simulink model "BbIb_parameter_estimation"  (R2022b)
settings: Solver=VariableStepAuto  StartTime=0.0  StopTime=25  MaxStep=0.005  RelTol=1e-3
values from neighbouring files (symbols this model uses):
  Bb = 0.00132333752617    [BbNew.mat]    (also in BbStiction.mat = 0.000317013532792; parameters.m = 0.000992; parametersDeadZone.m = 0.0001)
  Ib = 0.000954747737791    [IbNew.mat]    (also in IbStiction.mat = 0.000255111425973; parameters.m = 0.00072916; parametersDeadZone.m = 0.00036458)
  Ke = 0.089240515    [parameters.m]    (also in parametersDeadZone.m)
  Kt = 0.089240515    [parameters.m]    (also in parametersDeadZone.m)
  L = 0.0625    [parameters.m]    (also in parametersDeadZone.m)
  R = 5.0    (= 5)    [parameters.m]    (also in parametersDeadZone.m)
undefined symbols (not defined in the file or in its folder): sigbuilder_block
settings Model: Creator=47954  LastModifiedBy=47954

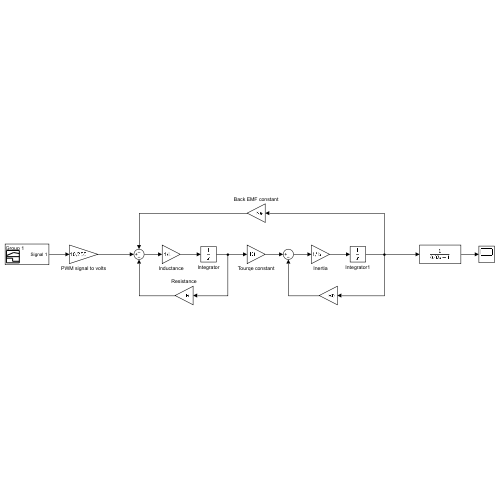
[thumbnail: Simulink's stored preview of the top-level diagram]
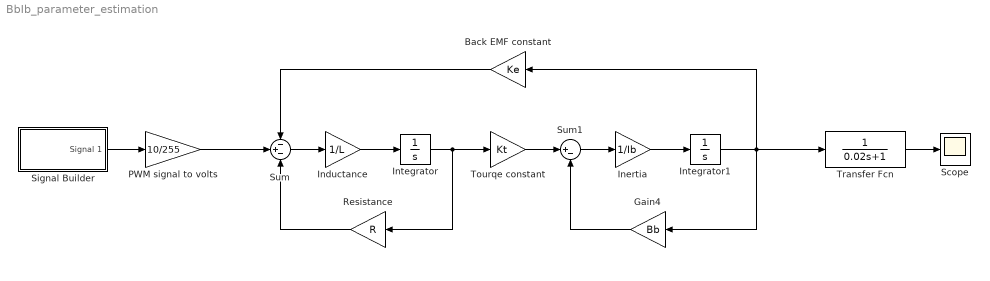
== system BbIb_parameter_estimation ==
  Back EMF constant : Gain  Gain=Ke
  Gain4 : Gain  Gain=Bb
  Inductance : Gain  Gain=1/L
  Inertia : Gain  Gain=1/Ib
  Integrator : Integrator
  Integrator1 : Integrator
  PWM signal to volts : Gain  Gain=10/255
  Resistance : Gain  Gain=R
  Scope : Scope
  Signal Builder : Subsystem  Tag=STV Subsys  LoadFcn=sigbuilder_block('load');  StartFcn=sigbuilder_block('start');  StopFcn=sigbuilder_block('stop');  ClipboardFcn=sigbuilder_block('clipboard');  mask(Sigbuilder block){tuvar=[0:10]}
      mask help: Simulink:masks:SigbuilderBlock_MD
      mask init:
      | if ~strcmp(get_param(bdroot(gcbh),'SimulationStatus'),'stopped') tuvar = sigbuilder_block('maskInit'); end
      settings: CopyFcn=sigbuilder_block('copy');  DeleteFcn=sigbuilder_block('delete');  ModelCloseFcn=sigbuilder_block('modelClose');  PreSaveFcn=sigbuilder_block('preSave');  PauseFcn=sigbuilder_block('pause');  ContinueFcn=sigbuilder_block('continue');  NameChangeFcn=sigbuilder_block('namechange');  OpenFcn=sigbuilder_block('open',[437.6 199.2 550.4 400 ]);  CloseFcn=sigbuilder_block('close');
      mask Display: plot(0, 0, 100, 100,[2, 2, 32, 32, 2], [68, 8, 8, 68, 68],[32, 2], [38, 38], [32, 19, 2],[53, 60, 44], [32, 17, 17, 2],[16, 16, 31, 31]);txt = getActiveGroup(gcbh);text(2, 100, txt,'verticalAlignment', 'top');
  Sum : Sum  Inputs=-+-
  Sum1 : Sum  Inputs=|+-
  Tourqe constant : Gain  Gain=Kt
  Transfer Fcn : TransferFcn  Denominator=[0.02 1]
  wires:
  Inductance/1 -> Integrator/1
  Integrator/1 -> Resistance/1, Tourqe constant/1
  Sum/1 -> Inductance/1
  Back EMF constant/1 -> Sum/1
  Resistance/1 -> Sum/3
  Gain4/1 -> Sum1/2
  Tourqe constant/1 -> Sum1/1
  Inertia/1 -> Integrator1/1
  Sum1/1 -> Inertia/1
  Integrator1/1 -> Transfer Fcn/1, Back EMF constant/1, Gain4/1
  Signal Builder/1(Signal 1) -> PWM signal to volts/1
  PWM signal to volts/1 -> Sum/2
  Transfer Fcn/1 -> Scope/1

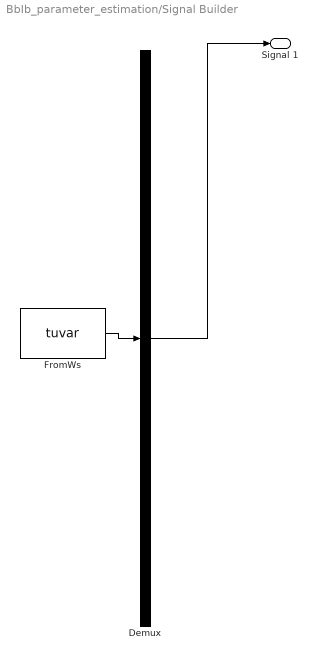
== system BbIb_parameter_estimation/Signal Builder ==
  Demux : Demux  Tag=STV Demux  Outputs=1
      settings: DisplayOption=none
  FromWs : FromWorkspace  Tag=STV FromWs  VariableName=tuvar
      SigBuilderData=|
      | common.afterFinalStr = 'Extrapolate'
      | common.sampleTime = 0
      | dataSet.timeRange = [0 25]
      | dataSet.name = 'Group 1'
      | sbobj.Groups.Name = 'Group 1'
      | sbobj.Groups.Signals.Name = 'Signal 1'
      | sbobj.Groups.Signals.XData = [0 5 5 10 10 15 15 20 20 25]
      | sbobj.Groups.Signals.YData = [-1 -1 100 100 0 0 -100 -100 0 0]
      | sbobj.Groups.TimeRange = [0 25]
  Signal 1 : Outport  Tag=STV Outport
  wires:
  FromWs/1 -> Demux/1
  Demux/1 -> Signal 1/1
